simulink model "differential_drive_robot_model_MFB"  (R2023a)
settings: Solver=FixedStepDiscrete  StartTime=0.0  StopTime=10.0  FixedStep=delta_time  RelTol=1e-3
model workspace (MAT data in the model file):
  TR = Simulink.Parameter
  TR.Value = 0.5
  TR.DataType = 'auto'
  TR.Complexity = 'real'
  TR.Dimensions = [1 1]
  delta_time = Simulink.Parameter
  delta_time.Value = 0.1
  delta_time.DataType = 'auto'
  delta_time.Complexity = 'real'
  delta_time.Dimensions = [1 1]
settings Model: Creator=tshintai  LastModifiedBy=fy153
settings OptimizationCC: DefaultParameterBehavior=Inlined  EnhancedBackFolding=on  PassReuseOutputArgsAs=Individual arguments  ZeroExternalMemoryAtStartup=off  ZeroInternalMemoryAtStartup=off  OptimizeBlockOrder=speed  DifferentSizesBufferReuse=on  OptimizationCustomize=off  EfficientTunableParamExpr=on
settings DebuggingCC: ParameterTunabilityLossMsg=error
settings SFSimCC: MATLABDynamicMemAlloc=off
settings RTWCC: Description=Embedded Coder  SystemTargetFile=ert.tlc  TemplateMakefile=ert_default_tmf  GenerateReport=on  LaunchReport=on  GenerateCodeMetricsReport=on
settings CodeAppCC: ForceParamTrailComments=on  IgnoreCustomStorageClasses=off  OperatorAnnotations=on  SimulinkDataObjDesc=on  SFDataObjDesc=on  InsertBlockDesc=on
settings ERTTargetCC: TargetLangStandard=C99 (ISO)  GenerateSampleERTMain=on  InlinedParameterPlacement=NonHierarchical  ERTCustomFileTemplate=example_file_process.tlc

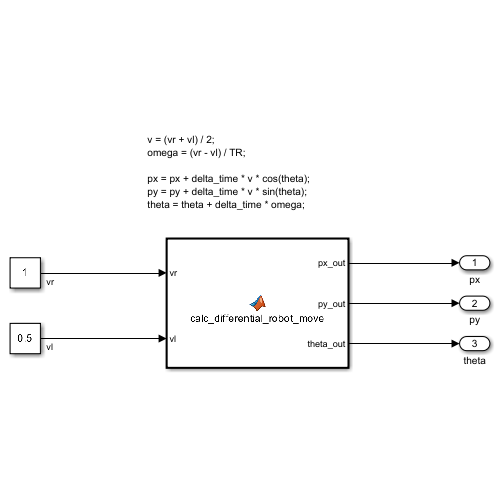
[thumbnail: Simulink's stored preview of the top-level diagram]
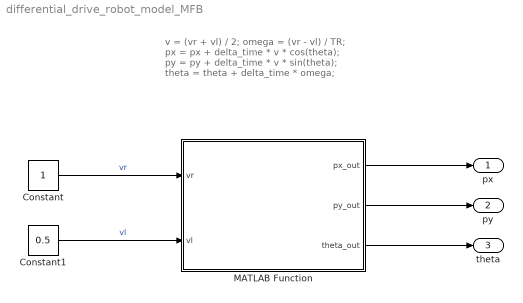
== system differential_drive_robot_model_MFB ==
  note: v = (vr + vl) / 2;
      | omega = (vr - vl) / TR;
      |
      | px = px + delta_time * v * cos(theta);
      | py = py + delta_time * v * sin(theta);
      | theta = theta + delta_time * omega;
  Constant : Constant
  Constant1 : Constant  Value=0.5
  MATLAB Function : MATLAB Function  TreatAsAtomicUnit=on
  px : Outport
  py : Outport  Port=2
  theta : Outport  Port=3
  wires:
  Constant1/1 -> MATLAB Function/2(vl)  "vl"
  Constant/1 -> MATLAB Function/1(vr)  "vr"
  MATLAB Function/1(px_out) -> px/1
  MATLAB Function/2(py_out) -> py/1
  MATLAB Function/3(theta_out) -> theta/1

== matlab function differential_drive_robot_model_MFB/MATLAB Function ==
  data: vr input; px_out output; vl input; py_out output; theta_out output; TR parameter; delta_time parameter
function [px_out, py_out, theta_out] = calc_differential_robot_move(vr, vl, TR, delta_time)

persistent px;
if isempty(px)
    px = 0;
end
persistent py;
if isempty(py)
    py = 0;
end
persistent theta;
if isempty(theta)
    theta = 0;
end
v = (vr + vl) / 2;
omega = (vr - vl) / TR;

px = px + delta_time * v * cos(theta);
py = py + delta_time * v * sin(theta);
theta = theta + delta_time * omega;

px_out = px;
py_out = py;
theta_out = theta;

end
